simulink model "Generic_13"  (R2022b)
settings: Solver=VariableStepAuto  StartTime=0.0  StopTime=10.0  RelTol=1e-3
values from neighbouring files (symbols this model uses):
  A = cell2mat(A_cell)    [MPCController1.m]    (also in MPC_Fmincon.m)
  B = cell2mat(B_cell)    [MPCController1.m]    (also in MPC_Fmincon.m)
  brake_select = ones(length(speed), length(steering_angle))    [TwoDLook_uptable.m]
  curvature = 0.000:0.001:1    [TwoDLook_uptable.m]
  m = 1600    [MPCController1.m]    (also in MPCController2.m; MPC_Fmincon.m)
  speed = 0:0.1:100    [TwoDLook_uptable.m]
undefined symbols (not defined in the file or in its folder): Amplifier, DiscIntNeverNeededParam, K_d_yawrate, K_dsteering, k_speed, k_stanley, kd, ki, kp, path_curvature
libraries: CarMaker4SL x121, simulink x12, cstblocks x7, autolibshared x1, mpcadaslib x1
(part 1 of 5)
settings Model: Creator=Admin  LastModifiedBy=Admin

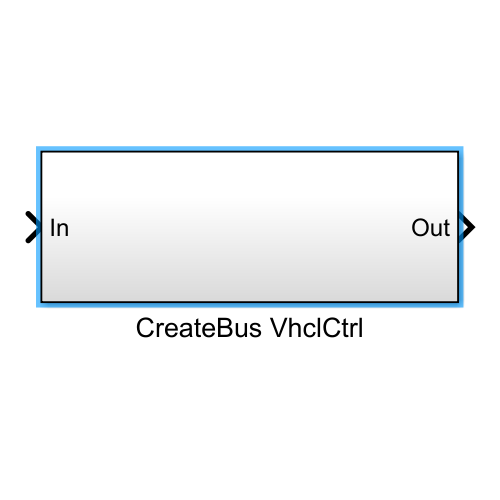
[thumbnail: Simulink's stored preview of the top-level diagram]
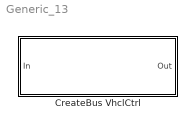
== system Generic_13 ==
  CreateBus VhclCtrl : Subsystem

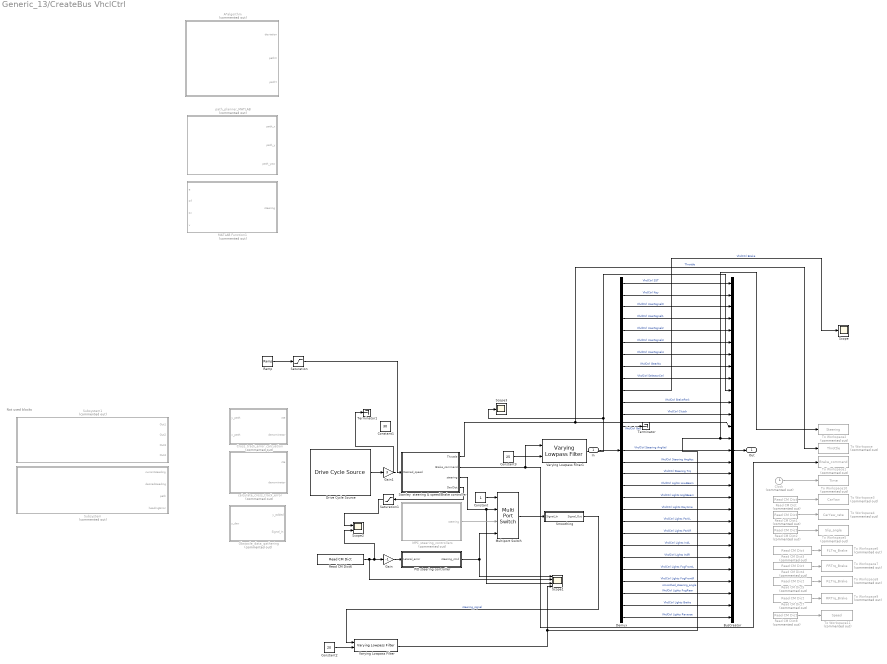
== system Generic_13/CreateBus VhclCtrl ==
  note: Not used blocks
  In : Inport
  A*algoithm : Subsystem  Commented=on
  BusCreator : BusCreator  Inputs=29
  Clock : Clock  Commented=on
  Constant : Constant
  Constant1 : Constant  Value=30
  Constant2 : Constant  Value=20
  Constant3 : Constant  Value=25
  Cross_track_error_calcuation : Subsystem  Commented=on
  Demux : Demux  Outputs=29
      settings: DisplayOption=none
  Drive Cycle Source : autolibshared/Drive Cycle Source  cycleVar=Artemis Motorway 150 kmph  fileVar=cycleFTP75.mat  tfinal="1068  seconds"  cycleRepeat=off  outAccPort=off  outGearPort=off  gearList=No gear data  t_wot1=5  xdot_woto=0  xdot_wot1=30  t_wot2=20  xdot_wot2=0  t_wotend=30  srcUnit=m/s  outUnit=m/s  srcAccUnit=m/s/s  outAccUnit=m/s^2  dt=1  aMode=2  faultOption=off  velBnd=2  velBndUnit=mph  inUnit=m/s  timeBnd=1  failOption=off  stopSim=off  maxFaultCnt=10  maxFaultTime=2  maxTotFaultTime=15  traceOption=off  dtTrace=1  traceWindow=10  lastDCname=Artemis Motorway 150 kmph  lastOutUnit=mph  lastDT=1  lastTB=1  lastSB=2  forceCalcBound=off
      settings: LibrarySourceBlock=vdynlib/Vehicle Scenarios/Drive Cycle and Maneuvers/Drive Cycle Source
  Gain : Gain  Gain=-1
  Gain1 : Gain  Gain=3
  MATLAB Function1 : MATLAB Function  Commented=on  TreatAsAtomicUnit=on
  MPC_steering_controllers : Subsystem  Commented=on
  Multiport Switch : MultiPortSwitch  SaturateOnIntegerOverflow=off  InputSameDT=off
  Obstacle_data_gathering : Subsystem  Commented=on
  PID steering controller : Subsystem
  Ramp : simulink/Sources/Ramp  slope=1  start=0  InitialOutput=0
  Read CM Dict : CarMaker4SL/Read CM Dict  Commented=on  xname=Car.Yaw  xsync=off  xstime=Continuous
  Read CM Dict1 : CarMaker4SL/Read CM Dict  Commented=on  xname=Car.YawRate  xsync=off  xstime=Continuous
  Read CM Dict2 : CarMaker4SL/Read CM Dict  Commented=on  xname=Sensor.SAngle.SS00.Ang  xsync=off  xstime=Continuous
  Read CM Dict3 : CarMaker4SL/Read CM Dict  Commented=on  xname=Vhcl.FL.Trq_Brake  xsync=off  xstime=Continuous
  Read CM Dict4 : CarMaker4SL/Read CM Dict  Commented=on  xname=Vhcl.FR.Trq_Brake  xsync=off  xstime=Continuous
  Read CM Dict5 : CarMaker4SL/Read CM Dict  Commented=on  xname=Vhcl.RL.Trq_Brake  xsync=off  xstime=Continuous
  Read CM Dict6 : CarMaker4SL/Read CM Dict  xname=Car.Road.Path.DevDist  xsync=off  xstime=Continuous
  Read CM Dict7 : CarMaker4SL/Read CM Dict  Commented=on  xname=Vhcl.RR.Trq_Brake  xsync=off  xstime=Continuous
  Read CM Dict8 : CarMaker4SL/Read CM Dict  Commented=on  xname=Vhcl.v  xsync=off  xstime=Continuous
  Saturation : Saturate  UpperLimit=66  LowerLimit=0
  Saturation1 : Saturate  UpperLimit=3  LowerLimit=-1
  Scope : Scope
  Scope1 : Scope  NumInputPorts=4
  Scope2 : Scope  NumInputPorts=2
  Scope3 : Scope
  Smoothing : Subsystem
  Stanley  steering & speed/Brake controller : Subsystem
  Subsystem : Subsystem  Commented=on
  Subsystem1 : Subsystem  Commented=on
  Terminator : Terminator
  Terminator1 : Terminator
  To Workspace : ToWorkspace  Commented=on  VariableName=Throttle  SampleTime=-1
      settings: Save2DSignal=2-D array (concatenate along first dimension)
  To Workspace1 : ToWorkspace  Commented=on  VariableName=Brake_command  SampleTime=-1
      settings: Save2DSignal=2-D array (concatenate along first dimension)
  To Workspace10 : ToWorkspace  Commented=on  VariableName=Time  SampleTime=-1
      settings: Save2DSignal=2-D array (concatenate along first dimension)
  To Workspace11 : ToWorkspace  Commented=on  VariableName=Speed  SampleTime=-1
      settings: Save2DSignal=2-D array (concatenate along first dimension)
  To Workspace2 : ToWorkspace  Commented=on  VariableName=Steering  SampleTime=-1
      settings: Save2DSignal=2-D array (concatenate along first dimension)
  To Workspace3 : ToWorkspace  Commented=on  VariableName=CarYaw  SampleTime=-1
      settings: Save2DSignal=2-D array (concatenate along first dimension)
  To Workspace4 : ToWorkspace  Commented=on  VariableName=CarYaw_rate  SampleTime=-1
      settings: Save2DSignal=2-D array (concatenate along first dimension)
  To Workspace5 : ToWorkspace  Commented=on  VariableName=Slip_angle  SampleTime=-1
      settings: Save2DSignal=2-D array (concatenate along first dimension)
  To Workspace6 : ToWorkspace  Commented=on  VariableName=FLTrq_Brake  SampleTime=-1
      settings: Save2DSignal=2-D array (concatenate along first dimension)
  To Workspace7 : ToWorkspace  Commented=on  VariableName=FRTrq_Brake  SampleTime=-1
      settings: Save2DSignal=2-D array (concatenate along first dimension)
  To Workspace8 : ToWorkspace  Commented=on  VariableName=RLTrq_Brake  SampleTime=-1
      settings: Save2DSignal=2-D array (concatenate along first dimension)
  To Workspace9 : ToWorkspace  Commented=on  VariableName=RRTrq_Brake  SampleTime=-1
      settings: Save2DSignal=2-D array (concatenate along first dimension)
  Varying Lowpass Filter : cstblocks/Linear Parameter Varying/Varying Lowpass Filter  N=1
  Varying Lowpass Filter1 : cstblocks/Linear Parameter Varying/Varying Lowpass Filter  N=1
  calculate_cross_track_error : Subsystem  Commented=on
  path_planner_MATLAB : Subsystem  Commented=on
  Out : Outport  VectorParamsAs1DForOutWhenUnconnected=off
  wires:
  Demux/2 -> BusCreator/2  "VhclCtrl Key"
  Demux/11 -> BusCreator/11  "VhclCtrl BrakePark"
  Demux/7 -> BusCreator/7  "VhclCtrl UserSignal4"
  Demux/5 -> BusCreator/5  "VhclCtrl UserSignal2"
  Demux/9 -> BusCreator/9  "VhclCtrl SelectorCtrl"
  In/1 -> Demux/1
  Demux/1 -> BusCreator/1  "VhclCtrl SST"
  Demux/3 -> BusCreator/3  "VhclCtrl UserSignal0"
  Demux/16 -> BusCreator/16  "VhclCtrl Steering AngAcc"
  Demux/4 -> BusCreator/4  "VhclCtrl UserSignal1"
  Demux/6 -> BusCreator/6  "VhclCtrl UserSignal3"
  Demux/8 -> BusCreator/8  "VhclCtrl GearNo"
  Demux/12 -> BusCreator/12  "VhclCtrl Clutch"
  Demux/15 -> BusCreator/15  "VhclCtrl Steering AngVel"
  Demux/17 -> BusCreator/17  "VhclCtrl Steering Trq"
  Demux/18 -> BusCreator/18  "VhclCtrl Lights LowBeam"
  Demux/19 -> BusCreator/19  "VhclCtrl Lights HighBeam"
  Demux/20 -> BusCreator/20  "VhclCtrl Lights Daytime"
  Demux/21 -> BusCreator/21  "VhclCtrl Lights ParkL"
  Demux/22 -> BusCreator/22  "VhclCtrl Lights ParkR"
  Demux/23 -> BusCreator/23  "VhclCtrl Lights IndL"
  Demux/24 -> BusCreator/24  "VhclCtrl Lights IndR"
  Demux/25 -> BusCreator/25  "VhclCtrl Lights FogFrontL"
  Demux/26 -> BusCreator/26  "VhclCtrl Lights FogFrontR"
  Demux/27 -> BusCreator/27  "VhclCtrl Lights FogRear"
  Demux/28 -> BusCreator/28  "VhclCtrl Lights Brake"
  Demux/29 -> BusCreator/29  "VhclCtrl Lights Reverse"
  BusCreator/1 -> Out/1
  Demux/13 -> Terminator/1  "VhclCtrl Gas"
  Stanley  steering & speed/Brake controller/3(steering) -> Scope1/3, Multiport Switch/2
  MPC_steering_controllers/1(steering) -> Multiport Switch/3
  Smoothing/1(Signal_Out) -> Varying Lowpass Filter/1  "steering_signal"
  Constant/1 -> Multiport Switch/1
  Stanley  steering & speed/Brake controller/1(Throttle) -> To Workspace/1, BusCreator/13  "Throttle"
  Gain/1 -> PID steering controller/1(Lateral_error)
  PID steering controller/1(steering_cmd) -> Multiport Switch/4, Scope1/1
  Stanley  steering & speed/Brake controller/4(DevDist) -> Saturation1/1
  Read CM Dict6/1 -> Gain/1, Scope2/2, Scope1/2
  Ramp/1 -> Saturation/1
  Constant2/1 -> Varying Lowpass Filter/2
  Varying Lowpass Filter/1 -> To Workspace2/1, BusCreator/14, Scope1/4  "smoothed_steering_angle"
  Multiport Switch/1 -> Smoothing/1(Signal_In)
  Drive Cycle Source/1 -> Gain1/1
  Read CM Dict/1 -> To Workspace3/1
  Read CM Dict1/1 -> To Workspace4/1
  Read CM Dict2/1 -> To Workspace5/1
  Read CM Dict3/1 -> To Workspace6/1
  Read CM Dict4/1 -> To Workspace7/1
  Read CM Dict5/1 -> To Workspace8/1
  Read CM Dict7/1 -> To Workspace9/1
  Clock/1 -> To Workspace10/1
  Read CM Dict8/1 -> To Workspace11/1
  Saturation1/1 -> Scope2/1
  Gain1/1 -> Terminator1/1
  Demux/10 -> Scope/1  "VhclCtrl Brake"
  Saturation/1 -> Stanley  steering & speed/Brake controller/1(Desired_speed)
  Stanley  steering & speed/Brake controller/2(Brake_command) -> Varying Lowpass Filter1/1, To Workspace1/1
  Constant3/1 -> Varying Lowpass Filter1/2
  Varying Lowpass Filter1/1 -> BusCreator/10, Scope3/1

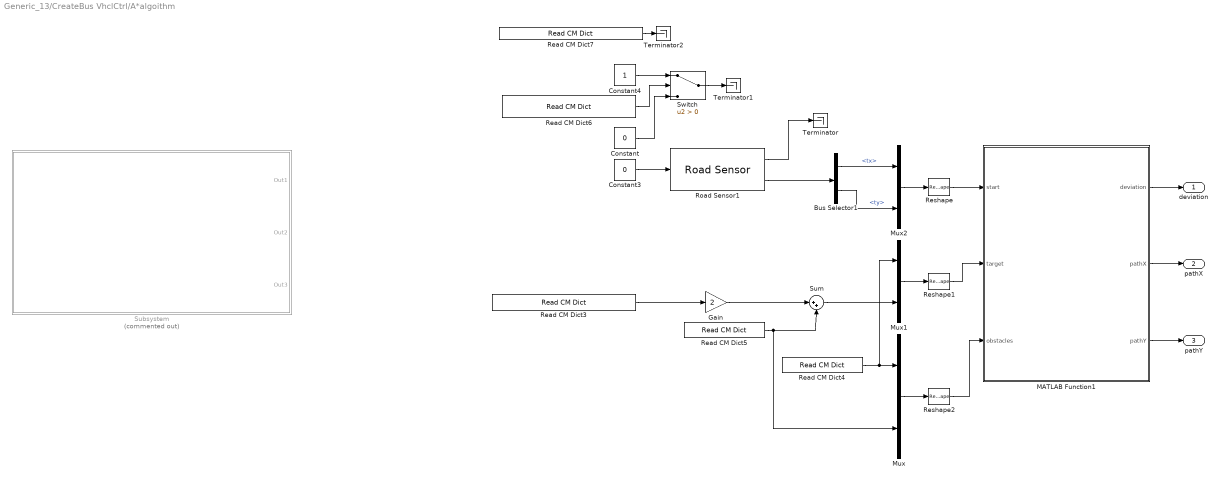
== system Generic_13/CreateBus VhclCtrl/A*algoithm ==
  Bus Selector1 : BusSelector  OutputSignals=Path.tx,Path.ty
  Constant : Constant  Value=0
  Constant3 : Constant  Value=0
  Constant4 : Constant
  Gain : Gain  Gain=2
  MATLAB Function1 : MATLAB Function  TreatAsAtomicUnit=on
  Mux : Mux  Inputs=2
  Mux1 : Mux  Inputs=2
  Mux2 : Mux  Inputs=2
  Read CM Dict3 : CarMaker4SL/Read CM Dict  xname=Sensor.Radar.VehSensor_6.Obj0.Length  xsync=off  xstime=Continuous
  Read CM Dict4 : CarMaker4SL/Read CM Dict  xname=Traffic.T00.tx  xsync=off  xstime=Continuous
  Read CM Dict5 : CarMaker4SL/Read CM Dict  xname=Traffic.T00.ty  xsync=off  xstime=Continuous
  Read CM Dict6 : CarMaker4SL/Read CM Dict  xname=Sensor.Radar.VehSensor_6.Obj0.ProbObst  xsync=off  xstime=Continuous
  Read CM Dict7 : CarMaker4SL/Read CM Dict  xname=Sensor.Radar.VehSensor_6.Obj0.Width  xsync=off  xstime=Continuous
  Reshape : Reshape  OutputDimensionality=Customize  OutputDimensions=[1,2]
  Reshape1 : Reshape  OutputDimensionality=Customize  OutputDimensions=[1,2]
  Reshape2 : Reshape  OutputDimensionality=Customize  OutputDimensions=[1,2]
  Road Sensor1 : CarMaker4SL/Sensors/Road Sensor  xname=0  xstime=Continuous
      settings: SourceProductName=CarMaker4SL
  Subsystem : Subsystem  Commented=on
  Sum : Sum  Inputs=|++
  Switch : Switch  Criteria=u2 > Threshold  SaturateOnIntegerOverflow=off  InputSameDT=off
  Terminator : Terminator
  Terminator1 : Terminator
  Terminator2 : Terminator
  deviation : Outport
  pathX : Outport  Port=2
  pathY : Outport  Port=3
  wires:
  Constant4/1 -> Switch/1
  Road Sensor1/2 -> Bus Selector1/1
  Road Sensor1/1 -> Terminator/1
  Read CM Dict4/1 -> Mux1/1, Mux/1
  Constant3/1 -> Road Sensor1/1
  Read CM Dict6/1 -> Switch/2
  Constant/1 -> Switch/3
  Read CM Dict3/1 -> Gain/1
  Gain/1 -> Sum/1
  Read CM Dict5/1 -> Sum/2, Mux/2
  Mux2/1 -> Reshape/1
  Bus Selector1/1 -> Mux2/1  "<tx>"
  Bus Selector1/2 -> Mux2/2  "<ty>"
  Sum/1 -> Mux1/2
  Mux1/1 -> Reshape1/1
  Mux/1 -> Reshape2/1
  Reshape/1 -> MATLAB Function1/1(start)
  Reshape1/1 -> MATLAB Function1/2(target)
  Reshape2/1 -> MATLAB Function1/3(obstacles)
  MATLAB Function1/1(deviation) -> deviation/1
  MATLAB Function1/2(pathX) -> pathX/1
  MATLAB Function1/3(pathY) -> pathY/1
  Switch/1 -> Terminator1/1
  Read CM Dict7/1 -> Terminator2/1

== system Generic_13/CreateBus VhclCtrl/Cross_track_error_calcuation ==
  y_path : Inport
  x_path : Inport  Port=2
  Cross_track_error_calcuation : MATLAB Function  TreatAsAtomicUnit=on
  Delay : Delay  DelayLength=1
  Delay1 : Delay  DelayLength=1
  Gain1 : Gain  Gain=-1
  Read CM Dict12 : CarMaker4SL/Read CM Dict  xname=Car.Gen.ty  xsync=off  xstime=Continuous
  Read CM Dict8 : CarMaker4SL/Read CM Dict  xname=Car.Gen.tx  xsync=off  xstime=Continuous
  cte : Outport
  denominator : Outport  Port=2
  wires:
  Read CM Dict12/1 -> Cross_track_error_calcuation/2(y_vehicle)
  x_path/1 -> Cross_track_error_calcuation/5(x2), Delay1/1
  y_path/1 -> Cross_track_error_calcuation/6(y2), Delay/1
  Cross_track_error_calcuation/2(denominator) -> denominator/1
  Read CM Dict8/1 -> Cross_track_error_calcuation/1(x_vehicle)
  Delay1/1 -> Cross_track_error_calcuation/3(x_point)
  Delay/1 -> Cross_track_error_calcuation/4(y_point)
  Cross_track_error_calcuation/1(cte) -> Gain1/1
  Gain1/1 -> cte/1

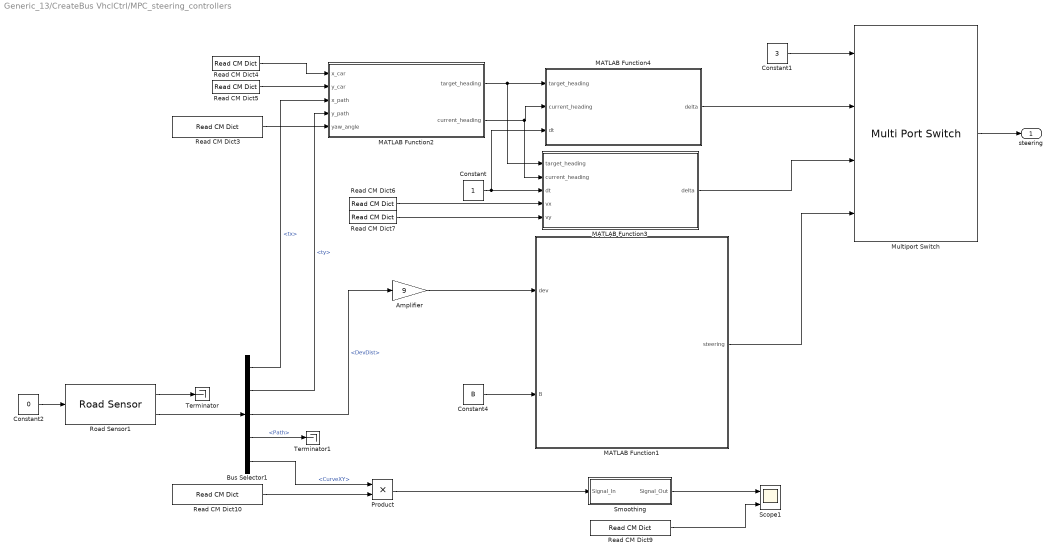
== system Generic_13/CreateBus VhclCtrl/MPC_steering_controllers ==
  Amplifier : Gain  Gain=9
  Bus Selector1 : BusSelector  OutputSignals=Path.tx,Path.ty,Path.DevDist,Path,Path.CurveXY
  Constant : Constant
  Constant1 : Constant  Value=3
  Constant2 : Constant  Value=0
  Constant4 : Constant  Value=B
  MATLAB Function1 : MATLAB Function  TreatAsAtomicUnit=on
  MATLAB Function2 : MATLAB Function  TreatAsAtomicUnit=on
  MATLAB Function3 : MATLAB Function  TreatAsAtomicUnit=on
  MATLAB Function4 : MATLAB Function  TreatAsAtomicUnit=on
  Multiport Switch : MultiPortSwitch  SaturateOnIntegerOverflow=off  InputSameDT=off
  Product : Product
  Read CM Dict10 : CarMaker4SL/Read CM Dict  xname=Vhcl.v  xsync=off  xstime=Continuous
  Read CM Dict3 : CarMaker4SL/Read CM Dict  xname=Vhcl.Yaw  xsync=off  xstime=Continuous
  Read CM Dict4 : CarMaker4SL/Read CM Dict  xname=Car.Con.tx  xsync=off  xstime=Continuous
  Read CM Dict5 : CarMaker4SL/Read CM Dict  xname=Car.Con.ty  xsync=off  xstime=Continuous
  Read CM Dict6 : CarMaker4SL/Read CM Dict  xname=Car.Con.vx_1  xsync=off  xstime=Continuous
  Read CM Dict7 : CarMaker4SL/Read CM Dict  xname=Car.Con.vy_1  xsync=off  xstime=Continuous
  Read CM Dict9 : CarMaker4SL/Read CM Dict  xname=Car.YawRate  xsync=off  xstime=Continuous
  Road Sensor1 : CarMaker4SL/Sensors/Road Sensor  xname=0  xstime=Continuous
      settings: SourceProductName=CarMaker4SL
  Scope1 : Scope  NumInputPorts=2
  Smoothing : Subsystem
  Terminator : Terminator
  Terminator1 : Terminator
  steering : Outport
  wires:
  Road Sensor1/1 -> Terminator/1
  Constant2/1 -> Road Sensor1/1
  Read CM Dict4/1 -> MATLAB Function2/1(x_car)
  Road Sensor1/2 -> Bus Selector1/1
  Read CM Dict3/1 -> MATLAB Function2/5(yaw_angle)
  Read CM Dict5/1 -> MATLAB Function2/2(y_car)
  Bus Selector1/5 -> Product/1  "<CurveXY>"
  Bus Selector1/1 -> MATLAB Function2/3(x_path)  "<tx>"
  Bus Selector1/2 -> MATLAB Function2/4(y_path)  "<ty>"
  Bus Selector1/3 -> Amplifier/1  "<DevDist>"
  Bus Selector1/4 -> Terminator1/1  "<Path>"
  Read CM Dict10/1 -> Product/2
  MATLAB Function2/1(target_heading) -> MATLAB Function4/1(target_heading), MATLAB Function3/1(target_heading)
  MATLAB Function3/1(delta) -> Multiport Switch/3
  MATLAB Function2/2(current_heading) -> MATLAB Function3/2(current_heading), MATLAB Function4/2(current_heading)
  Constant/1 -> MATLAB Function4/3(dt), MATLAB Function3/3(dt)
  Read CM Dict6/1 -> MATLAB Function3/4(vx)
  Read CM Dict7/1 -> MATLAB Function3/5(vy)
  Amplifier/1 -> MATLAB Function1/1(dev)
  Constant4/1 -> MATLAB Function1/2(B)
  Product/1 -> Smoothing/1(Signal_In)
  MATLAB Function4/1(delta) -> Multiport Switch/2
  MATLAB Function1/1(steering) -> Multiport Switch/4
  Smoothing/1(Signal_Out) -> Scope1/1
  Read CM Dict9/1 -> Scope1/2
  Multiport Switch/1 -> steering/1
  Constant1/1 -> Multiport Switch/1

== system Generic_13/CreateBus VhclCtrl/Obstacle_data_gathering ==
  y_dev : Inport
  Constant5 : Constant  Value=1.97
  Gain2 : Gain  Gain=-1
  MATLAB Function6 : MATLAB Function  TreatAsAtomicUnit=on
  MATLAB Function8 : MATLAB Function  TreatAsAtomicUnit=on
  Read CM Dict : CarMaker4SL/Read CM Dict  xname=Sensor.Object.VehSensor_5.relvTgt.NearPnt.ds.y  xsync=off  xstime=Continuous
  Read CM Dict1 : CarMaker4SL/Read CM Dict  xname=Car.Road.Path.DevDist  xsync=off  xstime=Continuous
  Read CM Dict11 : CarMaker4SL/Read CM Dict  xname=Sensor.Object.RadarL.relvTgt.NearPnt.ds.y  xsync=off  xstime=Continuous
  Read CM Dict13 : CarMaker4SL/Read CM Dict  xname=Sensor.Object.RadarL.Obj.T00.RefPnt.ds.x  xsync=off  xstime=Continuous
  Read CM Dict16 : CarMaker4SL/Read CM Dict  xname=Sensor.Object.VehSensor_4.relvTgt.NearPnt.ds.y  xsync=off  xstime=Continuous
  Read CM Dict17 : CarMaker4SL/Read CM Dict  xname=Sensor.Object.RadarL.relvTgt.NearPnt.ds.x  xsync=off  xstime=Continuous
  Scope : Scope  NumInputPorts=2
  Subsystem : Subsystem
  y_added : Outport
  Signal_In : Outport  Port=2
  wires:
  y_dev/1 -> MATLAB Function8/1(y_dev)
  Read CM Dict17/1 -> MATLAB Function6/7(x_distance_obj)
  Read CM Dict1/1 -> MATLAB Function6/1(path_dev)
  Constant5/1 -> MATLAB Function6/2(y_dev)
  Read CM Dict13/1 -> Scope/1, MATLAB Function8/3(distance), MATLAB Function6/6(distance)
  Read CM Dict11/1 -> MATLAB Function6/4(y_error_2)
  Read CM Dict16/1 -> MATLAB Function6/3(y_error3)
  Read CM Dict/1 -> MATLAB Function6/5(y_error), MATLAB Function8/2(data)
  MATLAB Function8/1(y_added) -> y_added/1
  MATLAB Function6/1(error) -> Gain2/1, Scope/2
  Gain2/1 -> Subsystem/1(In1)
  Subsystem/1(Signal_In) -> Signal_In/1

== system Generic_13/CreateBus VhclCtrl/PID steering controller ==
  Lateral_error : Inport
  Add : Sum  Inputs=+++
  Dervative : Subsystem
  Discrete-Time Integrator : DiscreteIntegrator  SampleTime=-1  ICPrevOutput=DiscIntNeverNeededParam  ICPrevScaledInput=DiscIntNeverNeededParam
  Gain : Gain  Gain=1.1
  Gain1 : Gain  Gain=0.9
  steering_cmd : Outport
  wires:
  Lateral_error/1 -> Gain1/1, Gain/1, Dervative/1(Error)
  Discrete-Time Integrator/1 -> Add/1
  Gain1/1 -> Discrete-Time Integrator/1
  Gain/1 -> Add/2
  Add/1 -> steering_cmd/1
  Dervative/1(Dervative term) -> Add/3

== system Generic_13/CreateBus VhclCtrl/Smoothing ==
  Signal_In : Inport
  Add : Sum  Inputs=++++
  Delay : Delay  InitialCondition=0.1
  Delay1 : Delay  DelayLength=4  InitialCondition=0.1
  Delay2 : Delay  DelayLength=5  InitialCondition=0.1
  Gain : Gain  Gain=0.35
  Gain1 : Gain  Gain=0.25
  Gain2 : Gain  Gain=0.25
  Gain3 : Gain  Gain=0.15
  Signal_Out : Outport  VectorParamsAs1DForOutWhenUnconnected=off
  wires:
  Gain1/1 -> Add/2
  Signal_In/1 -> Gain/1
  Delay/1 -> Gain1/1
  Gain/1 -> Add/1
  Delay1/1 -> Gain2/1
  Add/1 -> Delay2/1, Delay1/1, Delay/1, Signal_Out/1
  Gain2/1 -> Add/3
  Delay2/1 -> Gain3/1
  Gain3/1 -> Add/4

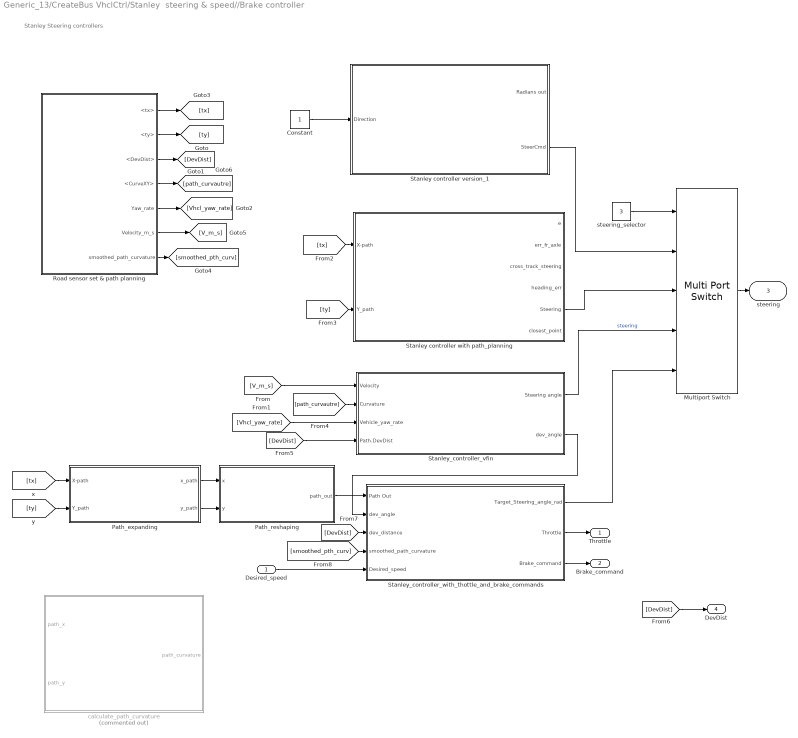
== system Generic_13/CreateBus VhclCtrl/Stanley  steering & speed//Brake controller ==
  note: Stanley Steering controllers
  Desired_speed : Inport
  " Path_expanding" : Subsystem
  Constant : Constant
  Multiport Switch : MultiPortSwitch  Inputs=4  SaturateOnIntegerOverflow=off  InputSameDT=off
  Path_reshaping : MATLAB Function  TreatAsAtomicUnit=on
  Road sensor set & path planning : Subsystem  Variant=on  VariantControlMode=label  VariantControl=Choice  LabelModeActiveChoice=Choice
  Stanley controller version_1 : Subsystem  Variant=on  VariantControlMode=label  VariantControl=Choice  LabelModeActiveChoice=Choice
  Stanley controller with path_planning : Subsystem  Variant=on  VariantControlMode=label  VariantControl=Choice  LabelModeActiveChoice=Choice
  Stanley_controller_vfin : Subsystem  Variant=on  VariantControlMode=label  VariantControl=Choice  LabelModeActiveChoice=Choice
  Stanley_controller_with_thottle_and_brake_commands : Subsystem
  calculate_path_curvature : Subsystem  Commented=on  Variant=on  VariantControlMode=label  VariantControl=Choice  LabelModeActiveChoice=Choice
  steering_selector : Constant  Value=3
  Throttle : Outport
  Brake_command : Outport  Port=2
  steering : Outport  Port=3
  DevDist : Outport  Port=4
  wires:
  [tx] -> " Path_expanding"/1(X-path)
  [ty] -> " Path_expanding"/2(Y_path)
  [tx] -> Stanley controller with path_planning/1(X-path)
  [ty] -> Stanley controller with path_planning/2(Y_path)
  Road sensor set & path planning/1(<tx>) -> [tx]
  Road sensor set & path planning/2(<ty>) -> [ty]
  Road sensor set & path planning/3(<DevDist>) -> [DevDist]
  Road sensor set & path planning/4(<CurveXY>) -> [path_curvautre]
  Road sensor set & path planning/5(Yaw_rate) -> [Vhcl_yaw_rate]
  [path_curvautre] -> Stanley_controller_vfin/2(Curvature)
  Stanley_controller_vfin/1(Steering angle) -> Multiport Switch/4  "steering"
  Constant/1 -> Stanley controller version_1/1(Direction)
  steering_selector/1 -> Multiport Switch/1
  Stanley controller version_1/2(SteerCmd) -> Multiport Switch/2
  Stanley controller with path_planning/5(Steering) -> Multiport Switch/3
  Path_reshaping/1(path_out) -> Stanley_controller_with_thottle_and_brake_commands/1(Path Out)
  Stanley_controller_vfin/2(dev_angle) -> Stanley_controller_with_thottle_and_brake_commands/2(dev_angle)
  " Path_expanding"/1(x_path) -> Path_reshaping/1(x)
  " Path_expanding"/2(y_path) -> Path_reshaping/2(y)
  Stanley_controller_with_thottle_and_brake_commands/2(Throttle) -> Throttle/1
  Stanley_controller_with_thottle_and_brake_commands/3(Brake_command) -> Brake_command/1
  Stanley_controller_with_thottle_and_brake_commands/1(Target_Steering_angle_rad) -> Multiport Switch/5
  [V_m_s] -> Stanley_controller_vfin/1(Velocity)
  [Vhcl_yaw_rate] -> Stanley_controller_vfin/3(Vehicle_yaw_rate)
  [DevDist] -> Stanley_controller_vfin/4(Path.DevDist)
  Road sensor set & path planning/6(Velocity_m_s) -> [V_m_s]
  [DevDist] -> DevDist/1
  Multiport Switch/1 -> steering/1
  [DevDist] -> Stanley_controller_with_thottle_and_brake_commands/3(dev_distance)
  Road sensor set & path planning/7(smoothed_path_curvature) -> [smoothed_pth_curv]
  [smoothed_pth_curv] -> Stanley_controller_with_thottle_and_brake_commands/4(smoothed_path_curvature)
  Desired_speed/1 -> Stanley_controller_with_thottle_and_brake_commands/5(Desired_speed)

== system Generic_13/CreateBus VhclCtrl/Subsystem ==
  " Path_expanding" : Subsystem  Commented=on
  Gain : Gain  Commented=on  Gain=-1
  MATLAB Function : MATLAB Function  Commented=on  TreatAsAtomicUnit=on
  MATLAB Function1 : MATLAB Function  Commented=on  TreatAsAtomicUnit=on
  Mux : Mux  Inputs=2
  Mux1 : Mux  Inputs=2
  PID steering controller : Subsystem  Commented=on
  Read CM Dict2 : CarMaker4SL/Read CM Dict  xname=Sensor.Road.VehSensor_0.Path.tx  xsync=off  xstime=Continuous
  Read CM Dict3 : CarMaker4SL/Read CM Dict  xname=Sensor.Road.VehSensor_0.Path.ty  xsync=off  xstime=Continuous
  Read CM Dict6 : CarMaker4SL/Read CM Dict  Commented=on  xname=Car.Road.Path.DevDist  xsync=off  xstime=Continuous
  Read CM Dict7 : CarMaker4SL/Read CM Dict  xname=Car.Road.tx  xsync=off  xstime=Continuous
  Read CM Dict9 : CarMaker4SL/Read CM Dict  xname=Car.Gen.ty  xsync=off  xstime=Continuous
  Reshape : Reshape  OutputDimensionality=Customize  OutputDimensions=[1,2]
  Reshape1 : Reshape  OutputDimensionality=Customize  OutputDimensions=[1,2]
  Subsystem3 : Subsystem  Commented=on
  currentHeading : Outport
  desiredHeading : Outport  Port=2
  path : Outport  Port=3
  headingError : Outport  Port=4
  wires:
  Read CM Dict2/1 -> Mux1/1, " Path_expanding"/1(X-path)
  Reshape/1 -> MATLAB Function/1(currentPosition)
  MATLAB Function/1(currentHeading) -> currentHeading/1
  Mux1/1 -> Reshape1/1
  Read CM Dict3/1 -> Mux1/2, " Path_expanding"/2(Y_path)
  Mux/1 -> Reshape/1
  MATLAB Function1/1(path) -> path/1
  " Path_expanding"/2(y_path) -> MATLAB Function1/2(y)
  " Path_expanding"/1(x_path) -> MATLAB Function1/1(x)
  Read CM Dict9/1 -> Mux/2
  MATLAB Function/2(desiredHeading) -> desiredHeading/1
  Reshape1/1 -> MATLAB Function/2(nextWaypoint)
  Read CM Dict7/1 -> Mux/1
  MATLAB Function/3(headingError) -> headingError/1
  Read CM Dict6/1 -> Gain/1
  Gain/1 -> PID steering controller/1(Lateral_error)

== system Generic_13/CreateBus VhclCtrl/Subsystem1 ==
  Delay : Delay  DelayLength=1
  Delay1 : Delay  DelayLength=1
  Gain : Gain  Gain=-2.3
  MATLAB Function : MATLAB Function  TreatAsAtomicUnit=on
  Mux : Mux  Inputs=2
  Mux1 : Mux  Inputs=2
  Mux2 : Mux  Inputs=2
  Read CM Dict2 : CarMaker4SL/Read CM Dict  xname=Sensor.Road.VehSensor_0.Path.tx  xsync=off  xstime=Continuous
  Read CM Dict3 : CarMaker4SL/Read CM Dict  xname=Sensor.Road.VehSensor_0.Path.ty  xsync=off  xstime=Continuous
  Read CM Dict4 : CarMaker4SL/Read CM Dict  xname=Car.Yaw  xsync=off  xstime=Continuous
  Read CM Dict7 : CarMaker4SL/Read CM Dict  xname=Car.Gen.tx  xsync=off  xstime=Continuous
  Read CM Dict9 : CarMaker4SL/Read CM Dict  xname=Car.Gen.ty  xsync=off  xstime=Continuous
  Reshape : Reshape  OutputDimensionality=Customize  OutputDimensions=[1,2]
  Reshape1 : Reshape  OutputDimensionality=Customize  OutputDimensions=[1,2]
  Reshape2 : Reshape  OutputDimensionality=Customize  OutputDimensions=[1,2]
  Out1 : Outport
  Out2 : Outport  Port=2
  Out3 : Outport  Port=3
  Out4 : Outport  Port=4
  wires:
  Read CM Dict7/1 -> MATLAB Function/1(vehicleX), Mux/1
  Read CM Dict2/1 -> MATLAB Function/3(pathX), Delay/1, Mux1/1
  Mux1/1 -> Reshape1/1
  Read CM Dict9/1 -> MATLAB Function/2(vehicleY), Mux/2
  MATLAB Function/1(deviationAngle) -> Gain/1
  Read CM Dict3/1 -> MATLAB Function/4(pathY), Delay1/1, Mux1/2
  Mux/1 -> Reshape/1
  Read CM Dict4/1 -> MATLAB Function/5(vehicleYaw)
  Mux2/1 -> Reshape2/1
  Reshape2/1 -> Out4/1
  Reshape/1 -> Out2/1
  Delay/1 -> Mux2/1
  Delay1/1 -> Mux2/2
  Gain/1 -> Out1/1
  Reshape1/1 -> Out3/1

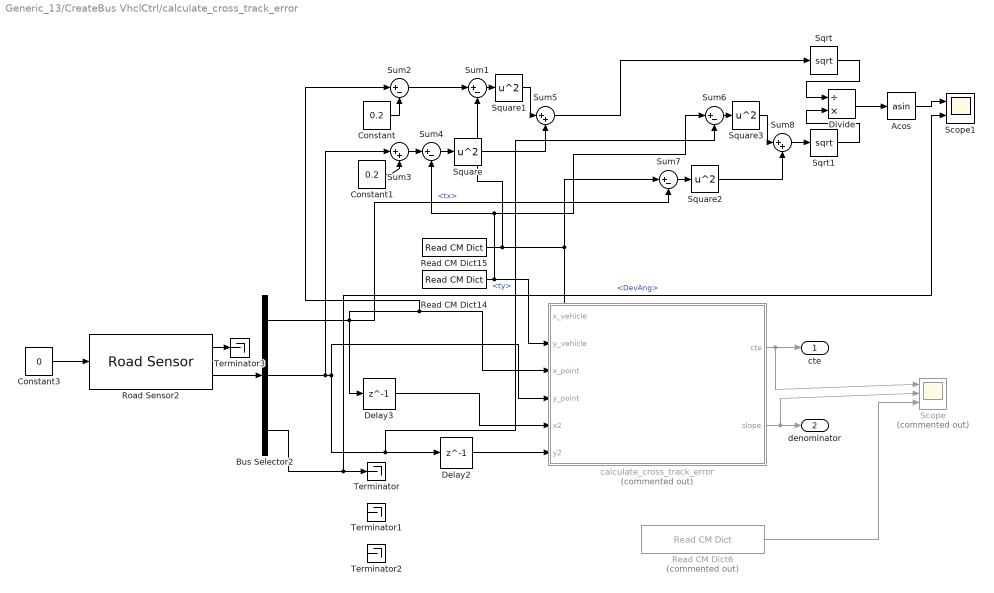
== system Generic_13/CreateBus VhclCtrl/calculate_cross_track_error ==
  Acos : Trigonometry  Operator=asin
  Bus Selector2 : BusSelector  OutputSignals=Path.tx,Path.ty,Path.DevAng
  Constant : Constant  Value=0.2
  Constant1 : Constant  Value=0.2
  Constant3 : Constant  Value=0
  Delay2 : Delay  DelayLength=1
  Delay3 : Delay  DelayLength=1
  Divide : Product  Inputs=/*
  Read CM Dict14 : CarMaker4SL/Read CM Dict  xname=Car.Gen.ty  xsync=off  xstime=Continuous
  Read CM Dict15 : CarMaker4SL/Read CM Dict  xname=Car.Gen.tx  xsync=off  xstime=Continuous
  Read CM Dict6 : CarMaker4SL/Read CM Dict  Commented=on  xname=Car.Road.Path.DevDist  xsync=off  xstime=Continuous
  Road Sensor2 : CarMaker4SL/Sensors/Road Sensor  xname=0  xstime=Continuous
      settings: SourceProductName=CarMaker4SL
  Scope : Scope  Commented=on  NumInputPorts=3
  Scope1 : Scope  NumInputPorts=2
  Sqrt : Sqrt
  Sqrt1 : Sqrt
  Square{,1..3} (4 alike) : Math  Operator=square
  Sum{1..2,4,6..7} (5 alike) : Sum  Inputs=|+-
  Sum3 : Sum  Inputs=|++
  Sum5 : Sum  Inputs=|++
  Sum8 : Sum  Inputs=|++
  Terminator{,1..3} (4 alike) : Terminator
  calculate_cross_track_error : MATLAB Function  Commented=on  TreatAsAtomicUnit=on
  cte : Outport
  denominator : Outport  Port=2
  wires:
  ? -> Terminator2/1  "<Path>"
  calculate_cross_track_error/2(slope) -> Scope/2, denominator/1
  Constant3/1 -> Road Sensor2/1
  Bus Selector2/2 -> Sum3/1, calculate_cross_track_error/4(y_point), Sum6/2, Delay2/1  "<ty>"
  Road Sensor2/1 -> Terminator3/1
  Road Sensor2/2 -> Bus Selector2/1
  Bus Selector2/1 -> Sum7/2, Sum2/1, calculate_cross_track_error/3(x_point), Delay3/1  "<tx>"
  Bus Selector2/3 -> Scope1/2, Terminator/1  "<DevAng>"
  ? -> Terminator1/1  "<CurveXY>"
  Read CM Dict15/1 -> Sum1/2, calculate_cross_track_error/1(x_vehicle), Sum7/1
  calculate_cross_track_error/1(cte) -> Scope/1, cte/1
  Read CM Dict6/1 -> Scope/3
  Delay2/1 -> calculate_cross_track_error/6(y2)
  Delay3/1 -> calculate_cross_track_error/5(x2)
  Constant/1 -> Sum2/2
  Constant1/1 -> Sum3/2
  Sum2/1 -> Sum1/1
  Sum3/1 -> Sum4/1
  Sum4/1 -> Square/1
  Sum1/1 -> Square1/1
  Square/1 -> Sum5/2
  Square1/1 -> Sum5/1
  Sum5/1 -> Sqrt/1
  Square2/1 -> Sum8/2
  Sum7/1 -> Square2/1
  Sum8/1 -> Sqrt1/1
  Square3/1 -> Sum8/1
  Sum6/1 -> Square3/1
  Read CM Dict14/1 -> calculate_cross_track_error/2(y_vehicle), Sum4/2, Sum6/1
  Sqrt/1 -> Divide/1
  Sqrt1/1 -> Divide/2
  Divide/1 -> Acos/1
  Acos/1 -> Scope1/1

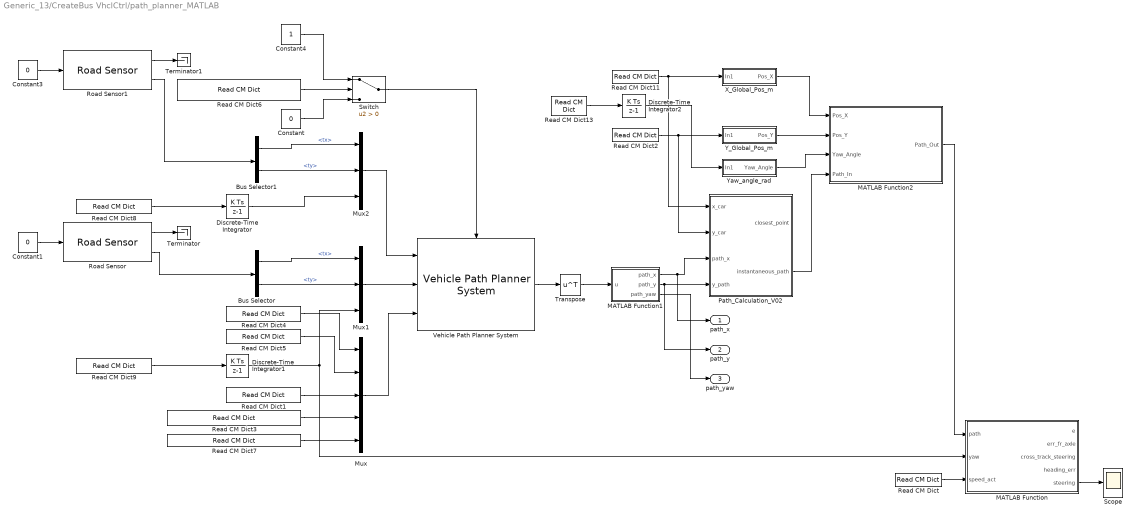
== system Generic_13/CreateBus VhclCtrl/path_planner_MATLAB ==
  Bus Selector : BusSelector  OutputSignals=Path.tx,Path.ty
  Bus Selector1 : BusSelector  OutputSignals=Path.tx,Path.ty
  Constant : Constant  Value=0
  Constant1 : Constant  Value=0
  Constant3 : Constant  Value=0
  Constant4 : Constant
  Discrete-Time Integrator : DiscreteIntegrator  SampleTime=-1  ICPrevOutput=DiscIntNeverNeededParam  ICPrevScaledInput=DiscIntNeverNeededParam
  Discrete-Time Integrator1 : DiscreteIntegrator  SampleTime=-1  ICPrevOutput=DiscIntNeverNeededParam  ICPrevScaledInput=DiscIntNeverNeededParam
  Discrete-Time Integrator2 : DiscreteIntegrator  SampleTime=-1  ICPrevOutput=DiscIntNeverNeededParam  ICPrevScaledInput=DiscIntNeverNeededParam
  MATLAB Function : MATLAB Function  TreatAsAtomicUnit=on
  MATLAB Function1 : MATLAB Function  TreatAsAtomicUnit=on
  MATLAB Function2 : MATLAB Function  TreatAsAtomicUnit=on
  Mux : Mux  Inputs=5
  Mux1 : Mux  Inputs=3
  Mux2 : Mux  Inputs=3
  Path_Calculation_V02 : MATLAB Function  TreatAsAtomicUnit=on
  Read CM Dict : CarMaker4SL/Read CM Dict  xname=Vhcl.v  xsync=off  xstime=Continuous
  Read CM Dict1 : CarMaker4SL/Read CM Dict  xname=Traffic.T00.rz  xsync=off  xstime=Continuous
  Read CM Dict11 : CarMaker4SL/Read CM Dict  xname=Car.Gen.tx  xsync=off  xstime=Continuous
  Read CM Dict13 : CarMaker4SL/Read CM Dict  xname=Car.YawRate  xsync=off  xstime=Continuous
  Read CM Dict2 : CarMaker4SL/Read CM Dict  xname=Car.Gen.ty  xsync=off  xstime=Continuous
  Read CM Dict3 : CarMaker4SL/Read CM Dict  xname=Sensor.Radar.VehSensor_6.Obj0.Length  xsync=off  xstime=Continuous
  Read CM Dict4 : CarMaker4SL/Read CM Dict  xname=Traffic.T00.tx  xsync=off  xstime=Continuous
  Read CM Dict5 : CarMaker4SL/Read CM Dict  xname=Traffic.T00.ty  xsync=off  xstime=Continuous
  Read CM Dict6 : CarMaker4SL/Read CM Dict  xname=Sensor.Radar.VehSensor_6.Obj0.ProbObst  xsync=off  xstime=Continuous
  Read CM Dict7 : CarMaker4SL/Read CM Dict  xname=Sensor.Radar.VehSensor_6.Obj0.Width  xsync=off  xstime=Continuous
  Read CM Dict8 : CarMaker4SL/Read CM Dict  xname=Car.YawRate  xsync=off  xstime=Continuous
  Read CM Dict9 : CarMaker4SL/Read CM Dict  xname=Car.YawRate  xsync=off  xstime=Continuous
  Road Sensor : CarMaker4SL/Sensors/Road Sensor  xname=0  xstime=Continuous
      settings: SourceProductName=CarMaker4SL
  Road Sensor1 : CarMaker4SL/Sensors/Road Sensor  xname=0  xstime=Continuous
      settings: SourceProductName=CarMaker4SL
  Scope : Scope
  Switch : Switch  Criteria=u2 > Threshold  SaturateOnIntegerOverflow=off  InputSameDT=off
  Terminator : Terminator
  Terminator1 : Terminator
  Transpose : Math  Operator=transpose
  Vehicle Path Planner System : mpcadaslib/Vehicle Path Planner System  egoLength=4.7  egoWidth=1.8  wheelbase=2.8  dist2Center=1.4  numObs=1  obsMat=zeros(1,5)  obs_ext=on  minDist=1  Ts=1  pPlanning=20  v_range=[-20,30]  v_ext=off  steer_range=[-pi/4,pi/4]  steer_ext=off  suboptimal=off  maxiter=200  output_exitflag=off
      settings: LibrarySourceBlock=mpclib/Automated Driving/Vehicle Path Planner System
  X_Global_Pos_m : Subsystem
  Y_Global_Pos_m : Subsystem
  Yaw_angle_rad : Subsystem
  path_x : Outport
  path_y : Outport  Port=2
  path_yaw : Outport  Port=3
  wires:
  Constant3/1 -> Road Sensor1/1
  Mux1/1 -> Vehicle Path Planner System/2
  Road Sensor/1 -> Terminator/1
  Road Sensor1/1 -> Terminator1/1
  Constant1/1 -> Road Sensor/1
  Bus Selector1/2 -> Mux2/2  "<ty>"
  Read CM Dict9/1 -> Discrete-Time Integrator1/1
  Road Sensor/2 -> Bus Selector/1
  Road Sensor1/2 -> Bus Selector1/1
  Read CM Dict8/1 -> Discrete-Time Integrator/1
  MATLAB Function2/1(Path_Out) -> MATLAB Function/1(path)
  Constant4/1 -> Switch/1
  Read CM Dict6/1 -> Switch/2
  Constant/1 -> Switch/3
  MATLAB Function1/1(path_x) -> Path_Calculation_V02/3(path_x), path_x/1
  Bus Selector1/1 -> Mux2/1  "<tx>"
  Discrete-Time Integrator/1 -> Mux2/3
  Bus Selector/1 -> Mux1/1  "<tx>"
  Bus Selector/2 -> Mux1/2  "<ty>"
  X_Global_Pos_m/1(Pos_X) -> MATLAB Function2/1(Pos_X)
  Read CM Dict4/1 -> Mux/1
  Read CM Dict5/1 -> Mux/2
  Read CM Dict11/1 -> Path_Calculation_V02/1(x_car), X_Global_Pos_m/1(In1)
  Discrete-Time Integrator1/1 -> MATLAB Function/2(yaw), Mux1/3
  Read CM Dict1/1 -> Mux/3
  Read CM Dict3/1 -> Mux/4
  Y_Global_Pos_m/1(Pos_Y) -> MATLAB Function2/2(Pos_Y)
  Read CM Dict7/1 -> Mux/5
  Transpose/1 -> MATLAB Function1/1(u)
  Switch/1 -> Vehicle Path Planner System/Enable
  Mux2/1 -> Vehicle Path Planner System/1
  Mux/1 -> Vehicle Path Planner System/3
  Vehicle Path Planner System/1 -> Transpose/1
  Read CM Dict13/1 -> Discrete-Time Integrator2/1
  Discrete-Time Integrator2/1 -> Yaw_angle_rad/1(In1)
  Read CM Dict2/1 -> Path_Calculation_V02/2(y_car), Y_Global_Pos_m/1(In1)
  MATLAB Function/5(steering) -> Scope/1
  MATLAB Function1/2(path_y) -> path_y/1, Path_Calculation_V02/4(y_path)
  MATLAB Function1/3(path_yaw) -> path_yaw/1
  Yaw_angle_rad/1(Yaw_Angle) -> MATLAB Function2/3(Yaw_Angle)
  Path_Calculation_V02/2(instantaneous_path) -> MATLAB Function2/4(Path_In)
  Read CM Dict/1 -> MATLAB Function/3(speed_act)

== system Generic_13/CreateBus VhclCtrl/A*algoithm/Subsystem ==
  Bus Selector : BusSelector  OutputSignals=Route.tx,Route.ty
  Constant : Constant  Value=0
  Constant1 : Constant  Value=0
  Read CM Dict : CarMaker4SL/Read CM Dict  xname=Sensor.Radar.VehSensor_6.Obj0.DistX  xsync=off  xstime=Continuous
  Read CM Dict1 : CarMaker4SL/Read CM Dict  xname=Sensor.Radar.VehSensor_6.Obj0.DistY  xsync=off  xstime=Continuous
  Read CM Dict3 : CarMaker4SL/Read CM Dict  xname=Sensor.Radar.VehSensor_6.Obj0.ProbObst  xsync=off  xstime=Continuous
  Road Sensor : CarMaker4SL/Sensors/Road Sensor  xname=0  xstime=Continuous
      settings: SourceProductName=CarMaker4SL
  Sum : Sum  Inputs=|++
  Sum1 : Sum  Inputs=|++
  Switch : Switch  Criteria=u2 > Threshold  SaturateOnIntegerOverflow=off  InputSameDT=off
  Switch1 : Switch  Criteria=u2 > Threshold  SaturateOnIntegerOverflow=off  InputSameDT=off
  Out1 : Outport
  Out2 : Outport  Port=2
  Out3 : Outport  Port=3
  wires:
  Read CM Dict1/1 -> Sum/1
  Sum/1 -> Switch/1
  Constant/1 -> Switch1/3, Switch/3
  Sum1/1 -> Switch1/1
  Switch/1 -> Out1/1
  Bus Selector/2 -> Sum1/1  "<ty>"
  Read CM Dict3/1 -> Switch1/2, Switch/2
  Read CM Dict/1 -> Sum1/2
  Road Sensor/2 -> Bus Selector/1
  Constant1/1 -> Road Sensor/1
  Bus Selector/1 -> Sum/2  "<tx>"
  Road Sensor/1 -> Out3/1
  Switch1/1 -> Out2/1

== system Generic_13/CreateBus VhclCtrl/MPC_steering_controllers/Smoothing ==
  Signal_In : Inport
  Add : Sum  Inputs=++++
  Delay : Delay  InitialCondition=0.1
  Delay1 : Delay  DelayLength=4  InitialCondition=0.1
  Delay2 : Delay  DelayLength=5  InitialCondition=0.1
  Gain : Gain  Gain=0.35
  Gain1 : Gain  Gain=0.25
  Gain2 : Gain  Gain=0.25
  Gain3 : Gain  Gain=0.15
  Signal_Out : Outport  VectorParamsAs1DForOutWhenUnconnected=off
  wires:
  Gain1/1 -> Add/2
  Signal_In/1 -> Gain/1
  Delay/1 -> Gain1/1
  Gain/1 -> Add/1
  Delay1/1 -> Gain2/1
  Add/1 -> Delay2/1, Delay1/1, Delay/1, Signal_Out/1
  Gain2/1 -> Add/3
  Delay2/1 -> Gain3/1
  Gain3/1 -> Add/4

== system Generic_13/CreateBus VhclCtrl/Obstacle_data_gathering/Subsystem ==
  In1 : Inport
  Add : Sum  Inputs=+++
  Derivative : Derivative
  Discrete-Time Integrator : DiscreteIntegrator  SampleTime=-1  ICPrevOutput=DiscIntNeverNeededParam  ICPrevScaledInput=DiscIntNeverNeededParam
  Gain : Gain  Gain=0.6
  Gain1 : Gain  Gain=1.2
  Gain2 : Gain  Gain=0.4
  Signal_In : Outport
  wires:
  Gain1/1 -> Discrete-Time Integrator/1
  Gain2/1 -> Derivative/1
  Discrete-Time Integrator/1 -> Add/1
  Derivative/1 -> Add/3
  Gain/1 -> Add/2
  In1/1 -> Gain/1, Gain2/1, Gain1/1
  Add/1 -> Signal_In/1

== system Generic_13/CreateBus VhclCtrl/PID steering controller/Dervative ==
  Error : Inport
  Discrete Derivative : simulink/Discrete/Discrete Derivative  gainval=1.0  ICPrevScaledInput=0.01  OutMin=[]  OutMax=[]  OutDataType=fixdt(1, 16)  OutScaling=2^-10  DoSatur=off
  Gain2 : Gain  Gain=0.4
  Dervative term : Outport
  wires:
  Error/1 -> Gain2/1
  Gain2/1 -> Discrete Derivative/1
  Discrete Derivative/1 -> Dervative term/1

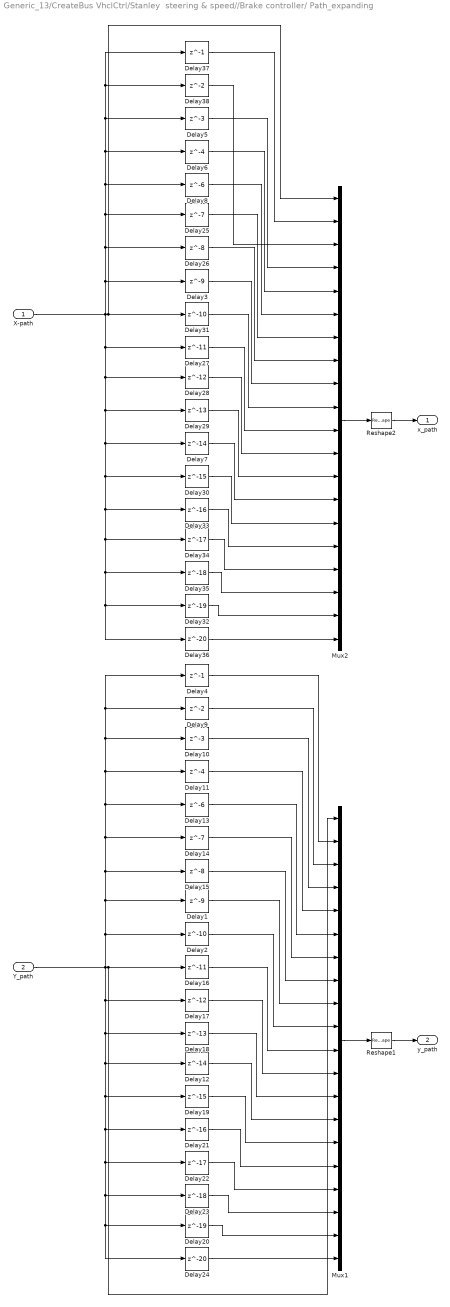
== system Generic_13/CreateBus VhclCtrl/Stanley  steering & speed//Brake controller/ Path_expanding ==
  X-path : Inport
  Y_path : Inport  Port=2
  Delay1 : Delay  DelayLength=9
  Delay10 : Delay  DelayLength=3
  Delay11 : Delay  DelayLength=4
  Delay12 : Delay  DelayLength=14
  Delay13 : Delay  DelayLength=6
  Delay14 : Delay  DelayLength=7
  Delay15 : Delay  DelayLength=8
  Delay16 : Delay  DelayLength=11
  Delay17 : Delay  DelayLength=12
  Delay18 : Delay  DelayLength=13
  Delay19 : Delay  DelayLength=15
  Delay2 : Delay  DelayLength=10
  Delay20 : Delay  DelayLength=19
  Delay21 : Delay  DelayLength=16
  Delay22 : Delay  DelayLength=17
  Delay23 : Delay  DelayLength=18
  Delay24 : Delay  DelayLength=20
  Delay25 : Delay  DelayLength=7
  Delay26 : Delay  DelayLength=8
  Delay27 : Delay  DelayLength=11
  Delay28 : Delay  DelayLength=12
  Delay29 : Delay  DelayLength=13
  Delay3 : Delay  DelayLength=9
  Delay30 : Delay  DelayLength=15
  Delay31 : Delay  DelayLength=10
  Delay32 : Delay  DelayLength=19
  Delay33 : Delay  DelayLength=16
  Delay34 : Delay  DelayLength=17
  Delay35 : Delay  DelayLength=18
  Delay36 : Delay  DelayLength=20
  Delay37 : Delay  DelayLength=1
  Delay38 : Delay
  Delay4 : Delay  DelayLength=1
  Delay5 : Delay  DelayLength=3
  Delay6 : Delay  DelayLength=4
  Delay7 : Delay  DelayLength=14
  Delay8 : Delay  DelayLength=6
  Delay9 : Delay
  Mux1 : Mux  Inputs=20
  Mux2 : Mux  Inputs=20
  Reshape1 : Reshape  OutputDimensionality=Customize  OutputDimensions=[1,20]
  Reshape2 : Reshape  OutputDimensionality=Customize  OutputDimensions=[1,20]
  x_path : Outport
  y_path : Outport  Port=2
  wires:
  Delay12/1 -> Mux1/14
  X-path/1 -> Delay32/1, Delay36/1, Delay35/1, Delay34/1, Delay33/1, Delay30/1, Delay7/1, Delay29/1, Delay28/1, Delay27/1, Delay31/1, Mux2/1, Delay38/1, Delay37/1, Delay5/1, Delay6/1, Delay8/1, Delay25/1, Delay26/1, Delay3/1
  Delay25/1 -> Mux2/7
  Delay17/1 -> Mux1/12
  Y_path/1 -> Delay20/1, Delay24/1, Delay23/1, Delay22/1, Delay21/1, Delay19/1, Delay12/1, Delay18/1, Delay17/1, Mux1/1, Delay16/1, Delay4/1, Delay9/1, Delay10/1, Delay11/1, Delay13/1, Delay14/1, Delay15/1, Delay1/1, Delay2/1
  Delay5/1 -> Mux2/4
  Delay37/1 -> Mux2/2
  Delay6/1 -> Mux2/5
  Delay38/1 -> Mux2/3
  Delay20/1 -> Mux1/19
  Delay18/1 -> Mux1/13
  Delay8/1 -> Mux2/6
  Delay26/1 -> Mux2/8
  Delay3/1 -> Mux2/9
  Delay31/1 -> Mux2/10
  Delay27/1 -> Mux2/11
  Delay24/1 -> Mux1/20
  Delay28/1 -> Mux2/12
  Delay29/1 -> Mux2/13
  Delay7/1 -> Mux2/14
  Delay30/1 -> Mux2/15
  Delay33/1 -> Mux2/16
  Mux1/1 -> Reshape1/1
  Delay34/1 -> Mux2/17
  Delay35/1 -> Mux2/18
  Delay1/1 -> Mux1/9
  Delay32/1 -> Mux2/19
  Delay15/1 -> Mux1/8
  Delay36/1 -> Mux2/20
  Reshape1/1 -> y_path/1
  Delay4/1 -> Mux1/2
  Delay16/1 -> Mux1/11
  Delay9/1 -> Mux1/3
  Delay21/1 -> Mux1/16
  Delay10/1 -> Mux1/4
  Delay11/1 -> Mux1/5
  Delay13/1 -> Mux1/6
  Reshape2/1 -> x_path/1
  Delay14/1 -> Mux1/7
  Delay2/1 -> Mux1/10
  Delay19/1 -> Mux1/15
  Delay22/1 -> Mux1/17
  Delay23/1 -> Mux1/18
  Mux2/1 -> Reshape2/1

== system Generic_13/CreateBus VhclCtrl/Stanley  steering & speed//Brake controller/Road sensor set & path planning ==
  Road sensor set & path planning : Subsystem  VariantControl=Choice
  <tx> : Outport
  <ty> : Outport  Port=2
  <DevDist> : Outport  Port=3
  <CurveXY> : Outport  Port=4
  Yaw_rate : Outport  Port=5
  Velocity_m_s : Outport  Port=6
  smoothed_path_curvature : Outport  Port=7

== system Generic_13/CreateBus VhclCtrl/Stanley  steering & speed//Brake controller/Stanley controller version_1 ==
  Direction : Inport
  Stanley controller version_1 : Subsystem  VariantControl=Choice  ReferencedSubsystem=Stanley_controller_version_1
  Radians out : Outport
  SteerCmd : Outport  Port=2

== system Generic_13/CreateBus VhclCtrl/Stanley  steering & speed//Brake controller/Stanley controller with path_planning ==
  X-path : Inport
  Y_path : Inport  Port=2
  Stanley controller with path_planning : Subsystem  VariantControl=Choice
  e : Outport
  err_fr_axle : Outport  Port=2
  cross_track_steering : Outport  Port=3
  heading_err : Outport  Port=4
  Steering : Outport  Port=5
  closest_point : Outport  Port=6

== system Generic_13/CreateBus VhclCtrl/Stanley  steering & speed//Brake controller/Stanley_controller_vfin ==
  Velocity : Inport
  Curvature : Inport  Port=2
  Vehicle_yaw_rate : Inport  Port=3
  Path.DevDist : Inport  Port=4
  Stanley_controller_vfin : Subsystem  Variant=on  VariantControlMode=label  VariantControl=Choice  LabelModeActiveChoice=Choice
  Steering angle : Outport
  dev_angle : Outport  Port=2

== system Generic_13/CreateBus VhclCtrl/Stanley  steering & speed//Brake controller/Stanley_controller_with_thottle_and_brake_commands ==
  Path Out : Inport
  dev_angle : Inport  Port=2
  dev_distance : Inport  Port=3
  smoothed_path_curvature : Inport  Port=4
  Desired_speed : Inport  Port=5
  Abs : Abs  SaturateOnIntegerOverflow=off
  Abs1 : Abs  SaturateOnIntegerOverflow=off
  Constant : Constant
  Constant1 : Constant
  Constant5 : Constant  Value=2
  MPCLongitudianl_contorl : Subsystem
  Memory3 : Memory
  Memory4 : Memory
  Stanley steering + PID speed controller : Subsystem
  Terminator : Terminator
  Throttle_selector : MultiPortSwitch  Inputs=2  SaturateOnIntegerOverflow=off  InputSameDT=off
  Target_Steering_angle_rad : Outport
  Throttle : Outport  Port=2
  Brake_command : Outport  Port=3
  wires:
  dev_angle/1 -> [dev_angle]
  Memory4/1 -> Stanley steering + PID speed controller/2(<Vx_Global_m_s>)
  Constant/1 -> Abs/1
  [dev_angle] -> Stanley steering + PID speed controller/4(dev_angle)
  smoothed_path_curvature/1 -> MPCLongitudianl_contorl/1(smoothed_path_curvature)
  Stanley steering + PID speed controller/1(Steering_angle_rad) -> MPCLongitudianl_contorl/3(steering_angle), Target_Steering_angle_rad/1
  Constant1/1 -> Abs1/1
  Path Out/1 -> Stanley steering + PID speed controller/1(Path_out)
  Abs/1 -> Memory4/1
  Constant5/1 -> Throttle_selector/1
  Abs1/1 -> Memory3/1
  Memory3/1 -> Stanley steering + PID speed controller/3(<Vy_Global_m_s>)
  MPCLongitudianl_contorl/1(actual_velocity) -> Stanley steering + PID speed controller/5(<Actual_Velocity_Car_m_s>)  "actual_velocity"
  MPCLongitudianl_contorl/3(throttle) -> Throttle_selector/3  "throttle"
  MPCLongitudianl_contorl/2(Deisred_speed) -> Stanley steering + PID speed controller/6(Desired_speed)  "Deisred_speed"
  dev_distance/1 -> Stanley steering + PID speed controller/7(dev_distance)  "Dev_dis"
  Stanley steering + PID speed controller/3(Brake_command) -> Terminator/1
  Throttle_selector/1 -> Throttle/1
  Desired_speed/1 -> MPCLongitudianl_contorl/2(Desired_speed)
  MPCLongitudianl_contorl/4(Brake) -> Brake_command/1  "Brake_command"
  Stanley steering + PID speed controller/2(Throttle) -> Throttle_selector/2

== system Generic_13/CreateBus VhclCtrl/Stanley  steering & speed//Brake controller/calculate_path_curvature ==
  path_x : Inport
  path_y : Inport  Port=2
  calculate_path_curvature : ModelReference  ModelNameDialog=calculate_path_curvature  SimulationMode=Normal  VariantControl=Choice  ModelReferenceVersion=6.16
  path_curvature : Outport

== system Generic_13/CreateBus VhclCtrl/Subsystem/ Path_expanding ==
  X-path : Inport
  Y_path : Inport  Port=2
  Delay1 : Delay  DelayLength=9
  Delay10 : Delay  DelayLength=3
  Delay11 : Delay  DelayLength=4
  Delay13 : Delay  DelayLength=6
  Delay14 : Delay  DelayLength=7
  Delay15 : Delay  DelayLength=8
  Delay25 : Delay  DelayLength=7
  Delay26 : Delay  DelayLength=8
  Delay3 : Delay  DelayLength=9
  Delay37 : Delay  DelayLength=1
  Delay38 : Delay
  Delay4 : Delay  DelayLength=1
  Delay5 : Delay  DelayLength=3
  Delay6 : Delay  DelayLength=4
  Delay8 : Delay  DelayLength=6
  Delay9 : Delay
  Mux1 : Mux  Inputs=9
  Mux2 : Mux  Inputs=9
  Reshape1 : Reshape  OutputDimensionality=Customize  OutputDimensions=[1,9]
  Reshape2 : Reshape  OutputDimensionality=Customize  OutputDimensions=[1,9]
  x_path : Outport
  y_path : Outport  Port=2
  wires:
  X-path/1 -> Mux2/1, Delay38/1, Delay37/1, Delay5/1, Delay6/1, Delay8/1, Delay25/1, Delay26/1, Delay3/1
  Delay25/1 -> Mux2/7
  Y_path/1 -> Mux1/1, Delay4/1, Delay9/1, Delay10/1, Delay11/1, Delay13/1, Delay14/1, Delay15/1, Delay1/1
  Delay5/1 -> Mux2/4
  Delay37/1 -> Mux2/2
  Delay6/1 -> Mux2/5
  Delay38/1 -> Mux2/3
  Delay8/1 -> Mux2/6
  Delay26/1 -> Mux2/8
  Mux1/1 -> Reshape1/1
  Delay1/1 -> Mux1/9
  Delay15/1 -> Mux1/8
  Reshape1/1 -> y_path/1
  Delay4/1 -> Mux1/2
  Delay9/1 -> Mux1/3
  Delay10/1 -> Mux1/4
  Delay11/1 -> Mux1/5
  Delay13/1 -> Mux1/6
  Reshape2/1 -> x_path/1
  Delay14/1 -> Mux1/7
  Mux2/1 -> Reshape2/1
  Delay3/1 -> Mux2/9

== system Generic_13/CreateBus VhclCtrl/Subsystem/PID steering controller ==
  Lateral_error : Inport
  Add : Sum  Inputs=+++
  Derivative : Derivative
  Discrete-Time Integrator : DiscreteIntegrator  SampleTime=-1  ICPrevOutput=DiscIntNeverNeededParam  ICPrevScaledInput=DiscIntNeverNeededParam
  Gain : Gain  Gain=0.6
  Gain1 : Gain  Gain=0.9
  Gain2 : Gain  Gain=0.4
  steering_cmd : Outport
  wires:
  Lateral_error/1 -> Gain1/1, Gain/1, Gain2/1
  Discrete-Time Integrator/1 -> Add/1
  Gain2/1 -> Derivative/1
  Gain1/1 -> Discrete-Time Integrator/1
  Gain/1 -> Add/2
  Derivative/1 -> Add/3
  Add/1 -> steering_cmd/1

== system Generic_13/CreateBus VhclCtrl/Subsystem/Subsystem3 ==
  AND : Logic  IconShape=distinctive  AllPortsSameDT=off  OutDataTypeStr=boolean
  AND1 : Logic  IconShape=distinctive  AllPortsSameDT=off  OutDataTypeStr=boolean
  Clock{,2..6} (6 alike) : Clock
  Compare To Constant : simulink/Logic and Bit Operations/Compare To Constant  relop=>=  const=8  OutDataTypeStr=boolean
  Compare To Constant2 : simulink/Logic and Bit Operations/Compare To Constant  relop=>=  const=0.05  OutDataTypeStr=boolean
  Compare To Constant3 : simulink/Logic and Bit Operations/Compare To Constant  relop=<  const=4  OutDataTypeStr=boolean
  Compare To Constant5 : simulink/Logic and Bit Operations/Compare To Constant  relop=>  const=4  OutDataTypeStr=boolean
  Compare To Constant6 : simulink/Logic and Bit Operations/Compare To Constant  relop=<  const=8  OutDataTypeStr=boolean
  Gain : Gain  Gain=1.95
  Gain2 : Gain  Gain=2
  Gain4 : Gain  Gain=2.4
  Sum3 : Sum  Inputs=|+++
  Out1 : Outport
  Out2 : Outport  Port=2
  wires:
  Clock4/1 -> Out2/1
  Clock5/1 -> Compare To Constant5/1
  Clock6/1 -> Compare To Constant6/1
  Compare To Constant6/1 -> AND1/2
  Clock2/1 -> Compare To Constant2/1
  Clock3/1 -> Compare To Constant3/1
  Clock/1 -> Compare To Constant/1
  Compare To Constant5/1 -> AND1/1
  AND1/1 -> Gain4/1
  Compare To Constant2/1 -> AND/1
  Compare To Constant3/1 -> AND/2
  Compare To Constant/1 -> Gain/1
  AND/1 -> Gain2/1
  Gain/1 -> Sum3/2
  Gain4/1 -> Sum3/3
  Gain2/1 -> Sum3/1
  Sum3/1 -> Out1/1

== system Generic_13/CreateBus VhclCtrl/path_planner_MATLAB/X_Global_Pos_m ==
  In1 : Inport
  Pos_X : Outport  VectorParamsAs1DForOutWhenUnconnected=off
  wires:
  In1/1 -> Pos_X/1

== system Generic_13/CreateBus VhclCtrl/path_planner_MATLAB/Y_Global_Pos_m ==
  In1 : Inport
  Pos_Y : Outport  VectorParamsAs1DForOutWhenUnconnected=off
  wires:
  In1/1 -> Pos_Y/1

== system Generic_13/CreateBus VhclCtrl/path_planner_MATLAB/Yaw_angle_rad ==
  In1 : Inport
  Yaw_Angle : Outport  VectorParamsAs1DForOutWhenUnconnected=off
  wires:
  In1/1 -> Yaw_Angle/1
